simulink model "progetto_ese1_sim"  (R2023a)
settings: Solver=VariableStepAuto  StartTime=0.0  StopTime=10.0  RelTol=1e-3
values from neighbouring files (symbols this model uses):
  g = 9.81    [progetto_ese1_primo.m]
  Jx = .05    (= 0.05)    [progetto_ese1_primo.m]
  Jy = .05    (= 0.05)    [progetto_ese1_primo.m]
  Jz = .05    (= 0.05)    [progetto_ese1_primo.m]
  m = 1.4    [progetto_ese1_primo.m]
settings Model: Creator=USER  LastModifiedBy=USER

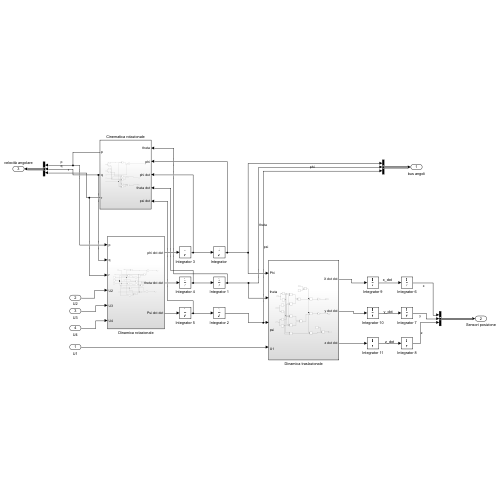
[thumbnail: Simulink's stored preview of the top-level diagram]
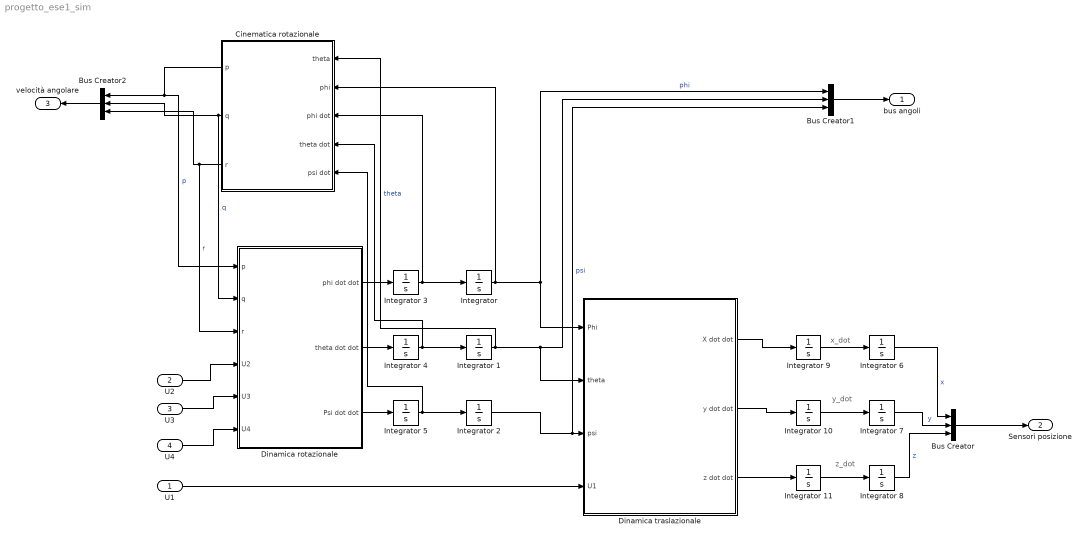
== system progetto_ese1_sim ==
  note: z_dot
  note: y_dot
  note: x_dot
  U1 : Inport
  U2 : Inport  Port=2
  U3 : Inport  Port=3
  U4 : Inport  Port=4
  Bus Creator : BusCreator  Inputs=3
  Bus Creator1 : BusCreator  Inputs=3
  Bus Creator2 : BusCreator  Inputs=3
  Cinematica rotazionale : Subsystem
  Dinamica rotazionale : Subsystem
  Dinamica traslazionale : Subsystem
  Integrator {,1..5,9..11} (9 alike) : Integrator
  Integrator 6 : Integrator  ContinuousStateAttributes=X_out
  Integrator 7 : Integrator  ContinuousStateAttributes=Y_out
  Integrator 8 : Integrator  ContinuousStateAttributes=Z_out
  bus angoli : Outport
  Sensori posizione : Outport  Port=2
  velocità angolare : Outport  Port=3
  wires:
  U4/1 -> Dinamica rotazionale/6(U4)
  U3/1 -> Dinamica rotazionale/5(U3)
  U2/1 -> Dinamica rotazionale/4(U2)
  Dinamica rotazionale/1(phi dot dot) -> Integrator 3/1
  Dinamica rotazionale/2(theta dot dot) -> Integrator 4/1
  Dinamica rotazionale/3(Psi dot dot) -> Integrator 5/1
  Integrator 3/1 -> Cinematica rotazionale/3(phi dot), "Integrator "/1
  Integrator 4/1 -> Cinematica rotazionale/4(theta dot), Integrator 1/1
  Integrator 5/1 -> Cinematica rotazionale/5(psi dot), Integrator 2/1
  U1/1 -> Dinamica traslazionale/4(U1)
  Integrator 2/1 -> Bus Creator1/3, Dinamica traslazionale/3(psi)  "psi"
  Integrator 1/1 -> Cinematica rotazionale/1(theta), Bus Creator1/2, Dinamica traslazionale/2(theta)  "theta"
  "Integrator "/1 -> Cinematica rotazionale/2(phi), Bus Creator1/1, Dinamica traslazionale/1(Phi)  "phi"
  Integrator 10/1 -> Integrator 7/1
  Integrator 9/1 -> Integrator 6/1
  Integrator 11/1 -> Integrator 8/1
  Dinamica traslazionale/1(X dot dot) -> Integrator 9/1
  Dinamica traslazionale/2(y dot dot) -> Integrator 10/1
  Dinamica traslazionale/3(z dot dot) -> Integrator 11/1
  Integrator 8/1 -> Bus Creator/3  "z"
  Integrator 7/1 -> Bus Creator/2  "y"
  Integrator 6/1 -> Bus Creator/1  "x"
  Bus Creator/1 -> Sensori posizione/1
  Bus Creator1/1 -> bus angoli/1
  Cinematica rotazionale/1(p) -> Dinamica rotazionale/1(p), Bus Creator2/1  "p"
  Cinematica rotazionale/2(q) -> Dinamica rotazionale/2(q), Bus Creator2/2  "q"
  Cinematica rotazionale/3(r) -> Dinamica rotazionale/3(r), Bus Creator2/3  "r"
  Bus Creator2/1 -> velocità angolare/1

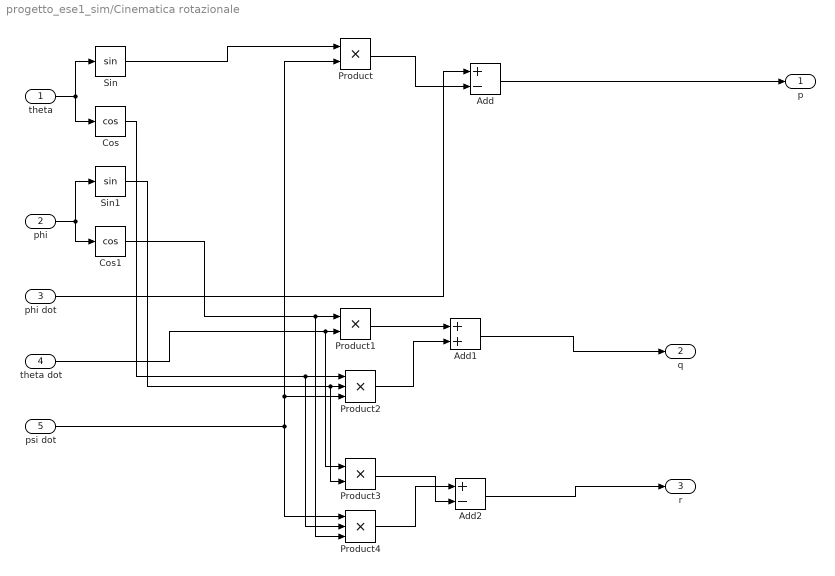
== system progetto_ese1_sim/Cinematica rotazionale ==
  theta : Inport
  phi : Inport  Port=2
  phi dot : Inport  Port=3
  theta dot : Inport  Port=4
  psi dot : Inport  Port=5
  Add : Sum  Inputs=+-
  Add1 : Sum
  Add2 : Sum  Inputs=+-
  Cos : Trigonometry  Operator=cos
  Cos1 : Trigonometry  Operator=cos
  Product : Product
  Product1 : Product
  Product2 : Product  Inputs=3
  Product3 : Product
  Product4 : Product  Inputs=3
  Sin : Trigonometry
  Sin1 : Trigonometry
  p : Outport
  q : Outport  Port=2
  r : Outport  Port=3
  wires:
  theta/1 -> Cos/1, Sin/1
  phi/1 -> Cos1/1, Sin1/1
  Sin/1 -> Product/1
  Add/1 -> p/1
  Product/1 -> Add/2
  psi dot/1 -> Product4/1, Product2/3, Product/2
  phi dot/1 -> Add/1
  Cos1/1 -> Product1/1, Product4/3
  theta dot/1 -> Product3/1, Product1/2
  Product1/1 -> Add1/1
  Product2/1 -> Add1/2
  Add1/1 -> q/1
  Sin1/1 -> Product3/2, Product2/2
  Cos/1 -> Product2/1, Product4/2
  Product4/1 -> Add2/1
  Product3/1 -> Add2/2
  Add2/1 -> r/1

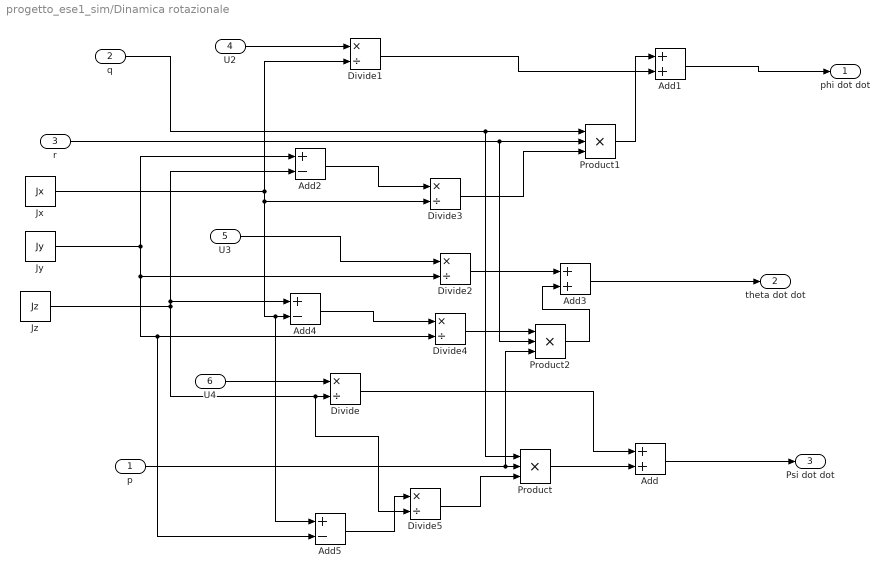
== system progetto_ese1_sim/Dinamica rotazionale ==
  p : Inport
  q : Inport  Port=2
  r : Inport  Port=3
  U2 : Inport  Port=4
  U3 : Inport  Port=5
  U4 : Inport  Port=6
  Add : Sum
  Add1 : Sum
  Add2 : Sum  Inputs=+-
  Add3 : Sum
  Add4 : Sum  Inputs=+-
  Add5 : Sum  Inputs=+-
  Divide{,1..5} (6 alike) : Product  Inputs=*/
  Jx : Constant  Value=Jx
  Jy : Constant  Value=Jy
  Jz : Constant  Value=Jz
  Product : Product  Inputs=3
  Product1 : Product  Inputs=3
  Product2 : Product  Inputs=3
  phi dot dot : Outport
  theta dot dot : Outport  Port=2
  Psi dot dot : Outport  Port=3
  wires:
  p/1 -> Product2/3, Product/2
  Product/1 -> Add/2
  Add/1 -> Psi dot dot/1
  U4/1 -> Divide/1
  Divide/1 -> Add/1
  U2/1 -> Divide1/1
  Divide1/1 -> Add1/2
  Add1/1 -> phi dot dot/1
  q/1 -> Product1/1, Product/1
  Product1/1 -> Add1/1
  r/1 -> Product1/2, Product2/2
  Jx/1 -> Divide3/2, Add5/1, Add4/2, Divide1/2
  Divide3/1 -> Product1/3
  Jy/1 -> Add5/2, Divide4/2, Divide2/2, Add2/1
  Add2/1 -> Divide3/1
  U3/1 -> Divide2/1
  Divide2/1 -> Add3/1
  Add3/1 -> theta dot dot/1
  Jz/1 -> Add4/1, Add2/2, Divide5/2, Divide/2
  Add4/1 -> Divide4/1
  Divide4/1 -> Product2/1
  Product2/1 -> Add3/2
  Divide5/1 -> Product/3
  Add5/1 -> Divide5/1

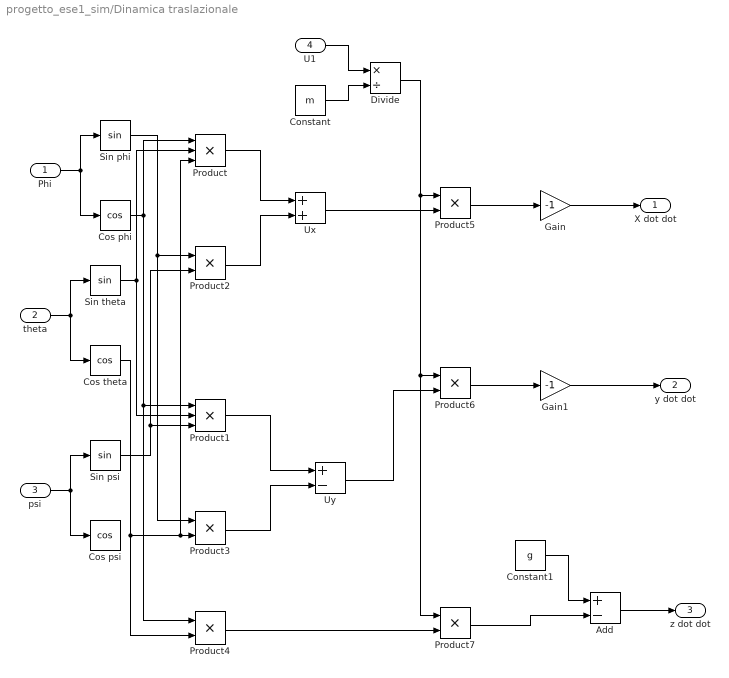
== system progetto_ese1_sim/Dinamica traslazionale ==
  Phi : Inport
  theta : Inport  Port=2
  psi : Inport  Port=3
  U1 : Inport  Port=4
  Add : Sum  Inputs=+-
  Constant : Constant  Value=m
  Constant1 : Constant  Value=g
  Cos phi : Trigonometry  Operator=cos
  Cos psi : Trigonometry  Operator=cos
  Cos theta : Trigonometry  Operator=cos
  Divide : Product  Inputs=*/
  Gain : Gain  Gain=-1
  Gain1 : Gain  Gain=-1
  Product : Product  Inputs=3
  Product1 : Product  Inputs=3
  Product{2..7} (6 alike) : Product
  Sin phi : Trigonometry
  Sin psi : Trigonometry
  Sin theta : Trigonometry
  Ux : Sum
  Uy : Sum  Inputs=+-
  X dot dot : Outport
  y dot dot : Outport  Port=2
  z dot dot : Outport  Port=3
  wires:
  Phi/1 -> Cos phi/1, Sin phi/1
  theta/1 -> Cos theta/1, Sin theta/1
  psi/1 -> Cos psi/1, Sin psi/1
  Sin phi/1 -> Product2/1, Product3/1
  Cos phi/1 -> Product1/1, Product4/1, Product/1
  Sin theta/1 -> Product1/2, Product/2
  Cos theta/1 -> Product/3, Product3/2, Product4/2
  Sin psi/1 -> Product1/3, Product2/2
  Product/1 -> Ux/1
  Product2/1 -> Ux/2
  Product1/1 -> Uy/1
  Product3/1 -> Uy/2
  Ux/1 -> Product5/2
  Product4/1 -> Product7/2
  Uy/1 -> Product6/2
  Constant/1 -> Divide/2
  U1/1 -> Divide/1
  Divide/1 -> Product7/1, Product6/1, Product5/1
  Product6/1 -> Gain1/1
  Product5/1 -> Gain/1
  Gain/1 -> X dot dot/1
  Gain1/1 -> y dot dot/1
  Product7/1 -> Add/2
  Constant1/1 -> Add/1
  Add/1 -> z dot dot/1
